simulink model "modelo2_fs_joy"  (Simulink 7.9)
settings: Solver=ode3  StartTime=0.0  StopTime=10  FixedStep=0.1  RelTol=1e-3
InitFcn:
  | modelo2Initialization
undefined symbols (not defined in the file or in its folder): Earth, WGS84
libraries: simulink_extras x2, aerolibfltsims x2, aerolibanimutils x2, aerolibtransform2 x1
settings Model: Creator=claus  LastModifiedBy=claus
settings SolverCC: ShapePreserveControl=EnableAll
settings OptimizationCC: SimCompilerOptimization=On  AccelVerboseBuild=on
settings ModelReferenceCC: EnableParallelModelReferenceBuilds=on

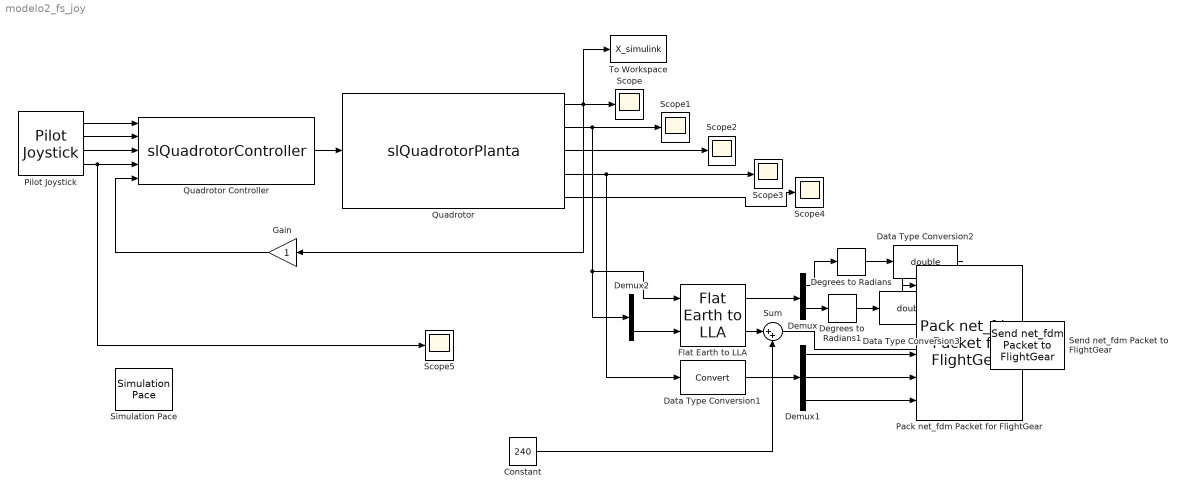
== system modelo2_fs_joy ==
  Constant : Constant  Value=240
  Data Type Conversion1 : DataTypeConversion
  Data Type Conversion2 : DataTypeConversion  OutDataTypeStr=double
  Data Type Conversion3 : DataTypeConversion  OutDataTypeStr=double
  Degrees to Radians : simulink_extras/Transformations/Degrees to Radians
  Degrees to Radians1 : simulink_extras/Transformations/Degrees to Radians
  Demux : Demux  Outputs=2
  Demux1 : Demux  Outputs=3
  Demux2 : Demux  Outputs=3
  Flat Earth to LLA : aerolibtransform2/Flat Earth to LLA  units=Metric (MKS)  ptype=Earth (WGS84)  F=1/298.257223563  R=6378137  LL0=[37.665543 -122.480847]  psi=0
  Gain : Gain
  Pack net_fdm Packet for FlightGear : aerolibfltsims/Pack net_fdm Packet for FlightGear  FlightGearVersion=v2.0  ShowPositionAttitudeInputs=on  ShowVelocityAccelerationInputs=off  ShowControlSurfacePositionInputs=off  ShowEngineFuelInputs=off  ShowLandingGearInputs=off  ShowEnvironmentInputs=off  SampleTime=-1
  Pilot Joystick : aerolibanimutils/Pilot Joystick  JoystickID=None  OutputConfiguration=FourAxis  SampleTime=0.1
  Quadrotor : M-S-Function  FunctionName=slQuadrotorPlanta
      mask init:
      | slQuadrotorPlantaInitialization
      mask Display:
      | port_label('output', 1, 'state x(1:12)')
      | port_label('output', 2, 'pos (I)')
      | port_label('output', 3, 'vel (B)')
      | port_label('output', 4, 'Euler (I) [Roll Pitch Yaw]')
      | port_label('output', 5, '\omega (B)')
      | port_label('input', 1, 'Control [f1 f2 f3 f4]')
  Quadrotor Controller : M-S-Function  FunctionName=slQuadrotorController
      mask Display:
      | port_label('output', 1, 'Control=[f1 f2 f3 f4]')
      | port_label('input', 1, 'Joystick roll')
      | port_label('input', 2, 'Joystick pitch')
      | port_label('input', 3, 'Joystick yaw')
      | port_label('input', 4, 'Joystick throttle')
      | port_label('input', 5, 'state x(1:12)')
  Scope{,1..5} (6 alike) : Scope
      Scope settings: TimeRange=1  YMin=-45  YMax=2.5
      Scope1 settings: TimeRange=1  YMin=-45  YMax=2.5
      Scope2 settings: TimeRange=1  YMin=-45  YMax=2.5  SaveName=ScopeData2
      Scope3 settings: TimeRange=1  YMin=-0.0025  YMax=0.03  SaveName=ScopeData3
      Scope4 settings: TimeRange=1  YMin=-0.01  YMax=0.11  SaveName=ScopeData4
      Scope5 settings: TimeRange=1  YMin=0.265  YMax=0.36  SaveName=ScopeData5
  Send net_fdm Packet to FlightGear : aerolibfltsims/Send net_fdm Packet to FlightGear  DestinationIpAddress=127.0.0.1  DestinationPort=5502  LocalIpPort=-1  varLen=off  SampleTime=-1
  Simulation Pace : aerolibanimutils/Simulation Pace  SimulationPace=1  SleepMode=MATLAB Thread  OutputPaceError=off  SampleTime=0.1
      settings: AttributesFormatString=%<SimulationPace> sec/sec
  Sum : Sum  Inputs=|++
  To Workspace : ToWorkspace  VariableName=X_simulink  SampleTime=-1  SaveFormat=Timeseries
  wires:
  Quadrotor Controller/1 -> Quadrotor/1
  Quadrotor/1 -> Scope/1, To Workspace/1, Gain/1
  Quadrotor/2 -> Demux2/1, Flat Earth to LLA/1, Scope1/1
  Quadrotor/3 -> Scope2/1
  Quadrotor/4 -> Data Type Conversion1/1, Scope3/1
  Quadrotor/5 -> Scope4/1
  Pack net_fdm Packet for FlightGear/1 -> Send net_fdm Packet to FlightGear/1
  Demux1/1 -> Pack net_fdm Packet for FlightGear/4
  Demux1/2 -> Pack net_fdm Packet for FlightGear/5
  Demux1/3 -> Pack net_fdm Packet for FlightGear/6
  Data Type Conversion1/1 -> Demux1/1
  Flat Earth to LLA/1 -> Demux/1
  Demux2/3 -> Flat Earth to LLA/2
  Degrees to Radians/1 -> Data Type Conversion2/1
  Degrees to Radians1/1 -> Data Type Conversion3/1
  Demux/1 -> Degrees to Radians/1
  Demux/2 -> Degrees to Radians1/1
  Data Type Conversion3/1 -> Pack net_fdm Packet for FlightGear/1
  Data Type Conversion2/1 -> Pack net_fdm Packet for FlightGear/2
  Flat Earth to LLA/2 -> Sum/1
  Constant/1 -> Sum/2
  Sum/1 -> Pack net_fdm Packet for FlightGear/3
  Pilot Joystick/1 -> Quadrotor Controller/1
  Pilot Joystick/2 -> Quadrotor Controller/2
  Pilot Joystick/3 -> Quadrotor Controller/3
  Pilot Joystick/4 -> Quadrotor Controller/4, Scope5/1
  Gain/1 -> Quadrotor Controller/5
